simulink model "model"  (R2019b)
settings: Solver=VariableStepAuto  StartTime=0.0  StopTime=100  RelTol=1e-3
libraries: simulink x1
settings Model: Creator=szymo  LastModifiedBy=szymo

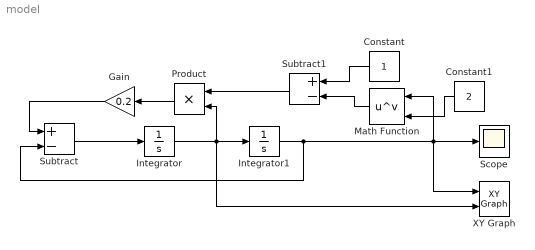
== system model ==
  Constant : Constant
  Constant1 : Constant  Value=2
  Gain : Gain  Gain=0.2
  Integrator : Integrator
  Integrator1 : Integrator  InitialCondition=0.1
  Math Function : Math  Operator=pow  SaturateOnIntegerOverflow=on
  Product : Product
  Scope : Scope
  Subtract : Sum  Inputs=+-
  Subtract1 : Sum  Inputs=+-
  XY Graph : simulink/Sinks/XY Graph  xmin=-3  xmax=3  ymin=-3  ymax=3  st=-1
  wires:
  Subtract/1 -> Integrator/1
  Integrator/1 -> XY Graph/2, Product/2, Integrator1/1
  Constant/1 -> Subtract1/1
  Math Function/1 -> Subtract1/2
  Subtract1/1 -> Product/1
  Product/1 -> Gain/1
  Gain/1 -> Subtract/1
  Constant1/1 -> Math Function/2
  Integrator1/1 -> XY Graph/1, Scope/1, Math Function/1, Subtract/2
